simulink subsystem "Regler"  (R2023b)
settings: Solver=VariableStepAuto  StartTime=0.0  StopTime=10.0  RelTol=1e-3
undefined symbols (not defined in the file or in its folder): K_p, T_n
settings Model: Creator=kilia  LastModifiedBy=mueller.chris-it22

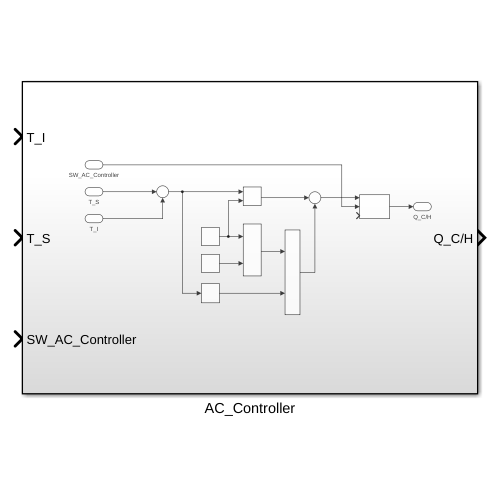
[thumbnail: Simulink's stored preview of the top-level diagram]
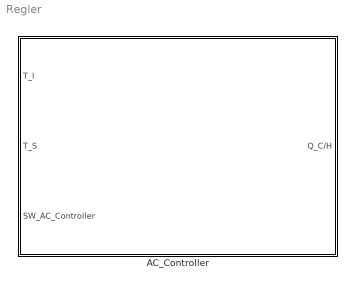
== system Regler ==
  AC_Controller : Subsystem

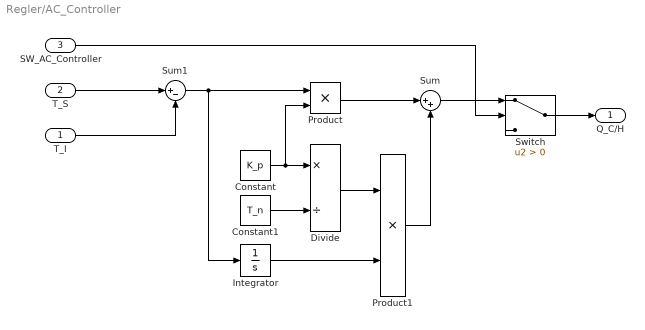
== system Regler/AC_Controller ==
  T_I : Inport
  T_S : Inport  Port=2
  SW_AC_Controller : Inport  Port=3
  Constant : Constant  Value=K_p
  Constant1 : Constant  Value=T_n
  Divide : Product  Inputs=*/
  Integrator : Integrator
  Product : Product
  Product1 : Product
  Sum : Sum  Inputs=|++
  Sum1 : Sum  Inputs=|+-
  Switch : Switch  Criteria=u2 > Threshold  SaturateOnIntegerOverflow=off  InputSameDT=off
  Q_C/H : Outport
  wires:
  Integrator/1 -> Product1/2
  Product/1 -> Sum/1
  Product1/1 -> Sum/2
  Sum1/1 -> Integrator/1, Product/1
  T_S/1 -> Sum1/1
  T_I/1 -> Sum1/2
  Constant/1 -> Product/2, Divide/1
  Constant1/1 -> Divide/2
  Divide/1 -> Product1/1
  Switch/1 -> Q_C/H/1
  Sum/1 -> Switch/1
  SW_AC_Controller/1 -> Switch/2
